simulink model "test_mex_in_slx_2018"  (R2024b)
settings: Solver=FixedStepAuto  StartTime=0.0  StopTime=10.0  FixedStep=1e-3  RelTol=1e-3
settings Model: Creator=39340  LastModifiedBy=39340
settings SolverCC: AlgebraicLoopSolver=TrustRegion
settings DebuggingCC: ArithmeticOperatorsInVariantConditions=warning
settings SFSimCC: CustomCodeUndefinedFunction=UseInterfaceOnly
settings RTWCC: GPUComputeCapability=3.5

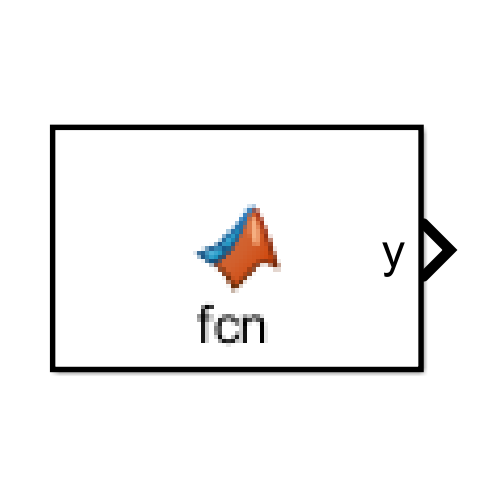
[thumbnail: Simulink's stored preview of the top-level diagram]
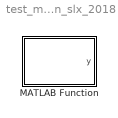
== system test_mex_in_slx_2018 ==
  MATLAB Function : MATLAB Function  TreatAsAtomicUnit=on

== matlab function test_mex_in_slx_2018/MATLAB Function ==
  data: y output
function y = fcn()

coder.extrinsic("net_predict_L_40k_mex")
out = net_predict_L_40k_mex(rand(1,10,6));

y = out(1,10,1);
